simulink model "downsample_demo_tests"  (R2019b)
settings: Solver=FixedStepDiscrete  StartTime=0  StopTime=100  RelTol=1e-3
libraries: dspsigops x6
settings Model: Creator=cyarp  LastModifiedBy=cyarp

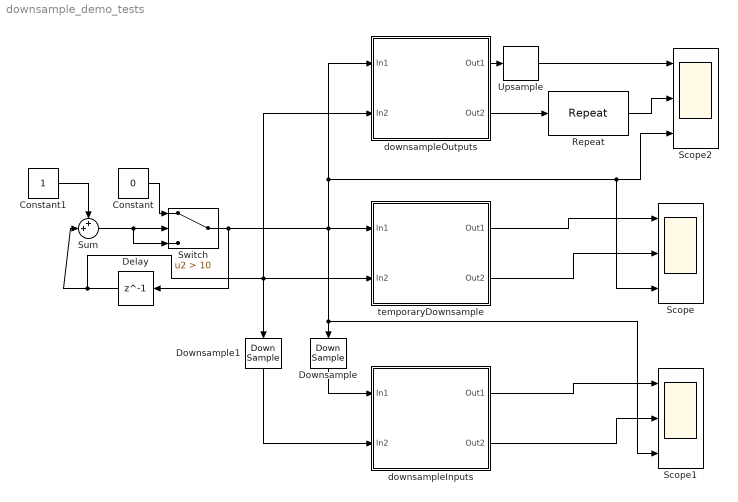
== system downsample_demo_tests ==
  Constant : Constant  Value=0  OutDataTypeStr=single
  Constant1 : Constant  OutDataTypeStr=single
  Delay : Delay  DelayLength=1  SampleTime=4
  Downsample : DownSample  N=4  RateOptions=Allow multirate processing
  Downsample1 : DownSample  N=4  RateOptions=Allow multirate processing
  Repeat : dspsigops/Repeat  N=4  InputProcessing=Columns as channels (frame based)  RateOptions=Allow multirate processing  ic=0  mode=Unused parameter value
      settings: SourceProductName=DSP System Toolbox
  Scope : Scope  NumInputPorts=3
  Scope1 : Scope  NumInputPorts=3
  Scope2 : Scope  NumInputPorts=3
  Sum : Sum  Inputs=++|
  Switch : Switch  Criteria=u2 > Threshold  Threshold=10
  Upsample : dspsigops/Upsample  N=4  phase=0  RateOptions=Allow multirate processing  ic=0  mode=Unused parameter value
  downsampleInputs : Subsystem
  downsampleOutputs : Subsystem
  temporaryDownsample : Subsystem
  wires:
  Delay/1 -> downsampleOutputs/2(In2), Downsample1/1, temporaryDownsample/2(In2), Sum/2
  Switch/1 -> Delay/1, temporaryDownsample/1(In1), downsampleOutputs/1(In1), Scope2/3, Scope/3, Scope1/3, Downsample/1
  Sum/1 -> Switch/2, Switch/3
  Constant/1 -> Switch/1
  Constant1/1 -> Sum/1
  temporaryDownsample/1(Out1) -> Scope/1
  temporaryDownsample/2(Out2) -> Scope/2
  downsampleInputs/1(Out1) -> Scope1/1
  downsampleInputs/2(Out2) -> Scope1/2
  Downsample1/1 -> downsampleInputs/2(In2)
  Downsample/1 -> downsampleInputs/1(In1)
  downsampleOutputs/1(Out1) -> Upsample/1
  downsampleOutputs/2(Out2) -> Repeat/1
  Upsample/1 -> Scope2/1
  Repeat/1 -> Scope2/2

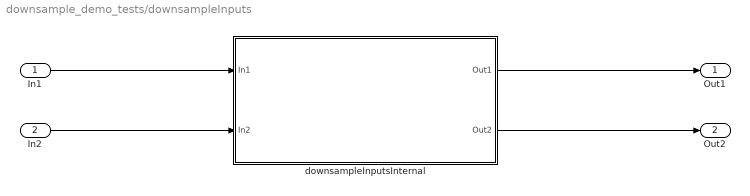
== system downsample_demo_tests/downsampleInputs ==
  In1 : Inport
  In2 : Inport  Port=2
  downsampleInputsInternal : Subsystem
  Out1 : Outport
  Out2 : Outport  Port=2
  wires:
  In1/1 -> downsampleInputsInternal/1(In1)
  In2/1 -> downsampleInputsInternal/2(In2)
  downsampleInputsInternal/1(Out1) -> Out1/1
  downsampleInputsInternal/2(Out2) -> Out2/1

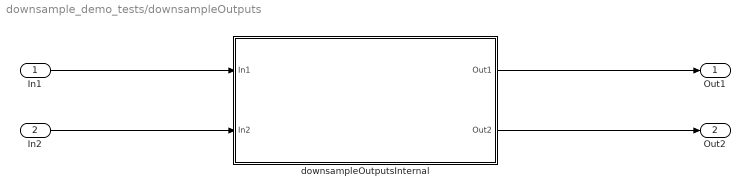
== system downsample_demo_tests/downsampleOutputs ==
  In1 : Inport
  In2 : Inport  Port=2
  downsampleOutputsInternal : Subsystem
  Out1 : Outport
  Out2 : Outport  Port=2
  wires:
  In1/1 -> downsampleOutputsInternal/1(In1)
  In2/1 -> downsampleOutputsInternal/2(In2)
  downsampleOutputsInternal/1(Out1) -> Out1/1
  downsampleOutputsInternal/2(Out2) -> Out2/1

== system downsample_demo_tests/temporaryDownsample ==
  In1 : Inport
  In2 : Inport  Port=2
  temporaryDownsampleInternal : Subsystem
  Out1 : Outport
  Out2 : Outport  Port=2
  wires:
  In1/1 -> temporaryDownsampleInternal/1(In1)
  In2/1 -> temporaryDownsampleInternal/2(In2)
  temporaryDownsampleInternal/1(Out1) -> Out1/1
  temporaryDownsampleInternal/2(Out2) -> Out2/1

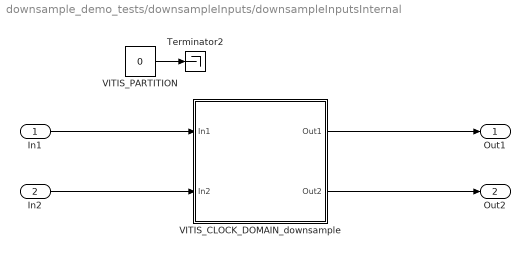
== system downsample_demo_tests/downsampleInputs/downsampleInputsInternal ==
  In1 : Inport
  In2 : Inport  Port=2
  Terminator2 : Terminator
  VITIS_CLOCK_DOMAIN_downsample : Subsystem
  VITIS_PARTITION : Constant  Value=0
  Out1 : Outport
  Out2 : Outport  Port=2
  wires:
  In1/1 -> VITIS_CLOCK_DOMAIN_downsample/1(In1)
  VITIS_CLOCK_DOMAIN_downsample/2(Out2) -> Out2/1
  In2/1 -> VITIS_CLOCK_DOMAIN_downsample/2(In2)
  VITIS_CLOCK_DOMAIN_downsample/1(Out1) -> Out1/1
  VITIS_PARTITION/1 -> Terminator2/1

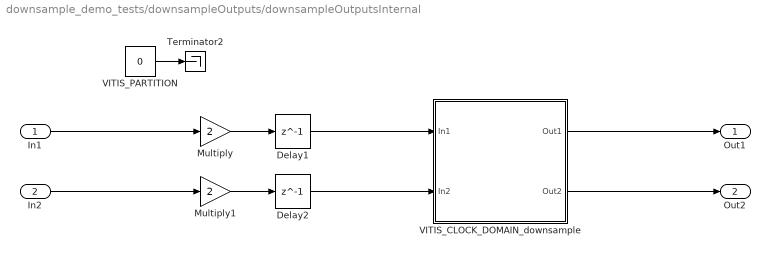
== system downsample_demo_tests/downsampleOutputs/downsampleOutputsInternal ==
  In1 : Inport
  In2 : Inport  Port=2
  Delay1 : Delay  DelayLength=1
  Delay2 : Delay  DelayLength=1
  Multiply : Gain  Gain=2
  Multiply1 : Gain  Gain=2
  Terminator2 : Terminator
  VITIS_CLOCK_DOMAIN_downsample : Subsystem
  VITIS_PARTITION : Constant  Value=0
  Out1 : Outport
  Out2 : Outport  Port=2
  wires:
  In1/1 -> Multiply/1
  In2/1 -> Multiply1/1
  Multiply1/1 -> Delay2/1
  Delay1/1 -> VITIS_CLOCK_DOMAIN_downsample/1(In1)
  VITIS_CLOCK_DOMAIN_downsample/2(Out2) -> Out2/1
  Multiply/1 -> Delay1/1
  Delay2/1 -> VITIS_CLOCK_DOMAIN_downsample/2(In2)
  VITIS_CLOCK_DOMAIN_downsample/1(Out1) -> Out1/1
  VITIS_PARTITION/1 -> Terminator2/1

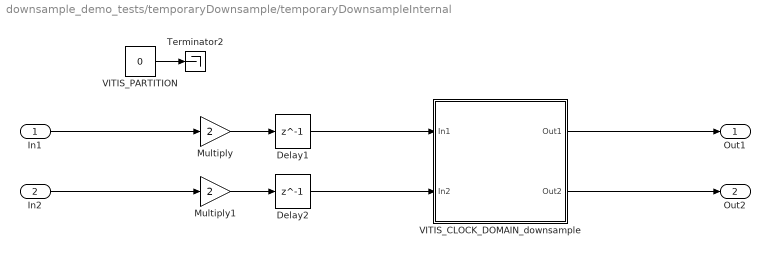
== system downsample_demo_tests/temporaryDownsample/temporaryDownsampleInternal ==
  In1 : Inport
  In2 : Inport  Port=2
  Delay1 : Delay  DelayLength=1
  Delay2 : Delay  DelayLength=1
  Multiply : Gain  Gain=2
  Multiply1 : Gain  Gain=2
  Terminator2 : Terminator
  VITIS_CLOCK_DOMAIN_downsample : Subsystem
  VITIS_PARTITION : Constant  Value=0
  Out1 : Outport
  Out2 : Outport  Port=2
  wires:
  In1/1 -> Multiply/1
  In2/1 -> Multiply1/1
  Multiply1/1 -> Delay2/1
  Delay1/1 -> VITIS_CLOCK_DOMAIN_downsample/1(In1)
  VITIS_CLOCK_DOMAIN_downsample/2(Out2) -> Out2/1
  Multiply/1 -> Delay1/1
  Delay2/1 -> VITIS_CLOCK_DOMAIN_downsample/2(In2)
  VITIS_CLOCK_DOMAIN_downsample/1(Out1) -> Out1/1
  VITIS_PARTITION/1 -> Terminator2/1

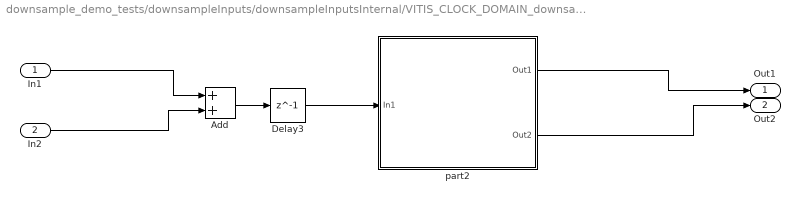
== system downsample_demo_tests/downsampleInputs/downsampleInputsInternal/VITIS_CLOCK_DOMAIN_downsample ==
  In1 : Inport
  In2 : Inport  Port=2
  Add : Sum
  Delay3 : Delay  DelayLength=1
  part2 : Subsystem
  Out1 : Outport
  Out2 : Outport  Port=2
  wires:
  Add/1 -> Delay3/1
  In2/1 -> Add/2
  In1/1 -> Add/1
  Delay3/1 -> part2/1(In1)
  part2/1(Out1) -> Out1/1
  part2/2(Out2) -> Out2/1

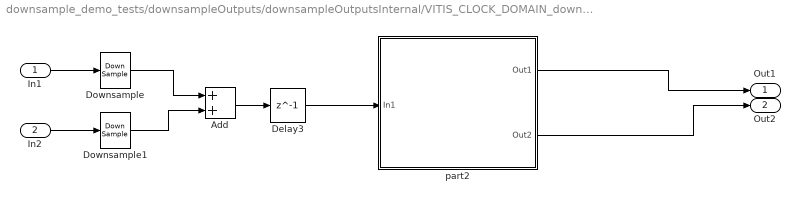
== system downsample_demo_tests/downsampleOutputs/downsampleOutputsInternal/VITIS_CLOCK_DOMAIN_downsample ==
  In1 : Inport
  In2 : Inport  Port=2
  Add : Sum
  Delay3 : Delay  DelayLength=1
  Downsample : DownSample  N=4  RateOptions=Allow multirate processing
  Downsample1 : DownSample  N=4  RateOptions=Allow multirate processing
  part2 : Subsystem
  Out1 : Outport
  Out2 : Outport  Port=2
  wires:
  Add/1 -> Delay3/1
  In2/1 -> Downsample1/1
  Downsample1/1 -> Add/2
  In1/1 -> Downsample/1
  Downsample/1 -> Add/1
  Delay3/1 -> part2/1(In1)
  part2/1(Out1) -> Out1/1
  part2/2(Out2) -> Out2/1

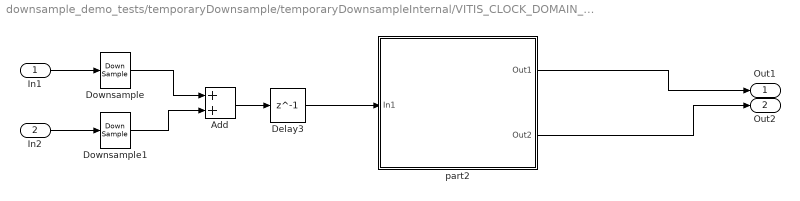
== system downsample_demo_tests/temporaryDownsample/temporaryDownsampleInternal/VITIS_CLOCK_DOMAIN_downsample ==
  In1 : Inport
  In2 : Inport  Port=2
  Add : Sum
  Delay3 : Delay  DelayLength=1
  Downsample : DownSample  N=4  RateOptions=Allow multirate processing
  Downsample1 : DownSample  N=4  RateOptions=Allow multirate processing
  part2 : Subsystem
  Out1 : Outport
  Out2 : Outport  Port=2
  wires:
  Add/1 -> Delay3/1
  In2/1 -> Downsample1/1
  Downsample1/1 -> Add/2
  In1/1 -> Downsample/1
  Downsample/1 -> Add/1
  Delay3/1 -> part2/1(In1)
  part2/1(Out1) -> Out1/1
  part2/2(Out2) -> Out2/1

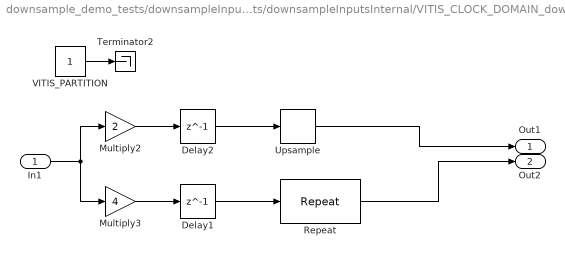
== system downsample_demo_tests/downsampleInputs/downsampleInputsInternal/VITIS_CLOCK_DOMAIN_downsample/part2 ==
  In1 : Inport
  Delay1 : Delay  DelayLength=1
  Delay2 : Delay  DelayLength=1
  Multiply2 : Gain  Gain=2
  Multiply3 : Gain  Gain=4
  Repeat : dspsigops/Repeat  N=4  InputProcessing=Columns as channels (frame based)  RateOptions=Allow multirate processing  ic=0  mode=Unused parameter value
      settings: SourceProductName=DSP System Toolbox
  Terminator2 : Terminator
  Upsample : dspsigops/Upsample  N=4  phase=0  RateOptions=Allow multirate processing  ic=0  mode=Unused parameter value
  VITIS_PARTITION : Constant
  Out1 : Outport
  Out2 : Outport  Port=2
  wires:
  Multiply2/1 -> Delay2/1
  Multiply3/1 -> Delay1/1
  Upsample/1 -> Out1/1
  Delay1/1 -> Repeat/1
  Delay2/1 -> Upsample/1
  Repeat/1 -> Out2/1
  In1/1 -> Multiply3/1, Multiply2/1
  VITIS_PARTITION/1 -> Terminator2/1

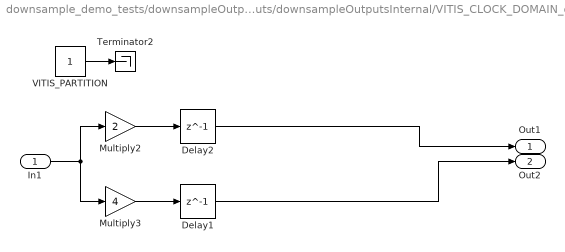
== system downsample_demo_tests/downsampleOutputs/downsampleOutputsInternal/VITIS_CLOCK_DOMAIN_downsample/part2 ==
  In1 : Inport
  Delay1 : Delay  DelayLength=1
  Delay2 : Delay  DelayLength=1
  Multiply2 : Gain  Gain=2
  Multiply3 : Gain  Gain=4
  Terminator2 : Terminator
  VITIS_PARTITION : Constant
  Out1 : Outport
  Out2 : Outport  Port=2
  wires:
  Multiply2/1 -> Delay2/1
  Multiply3/1 -> Delay1/1
  Delay2/1 -> Out1/1
  Delay1/1 -> Out2/1
  In1/1 -> Multiply3/1, Multiply2/1
  VITIS_PARTITION/1 -> Terminator2/1

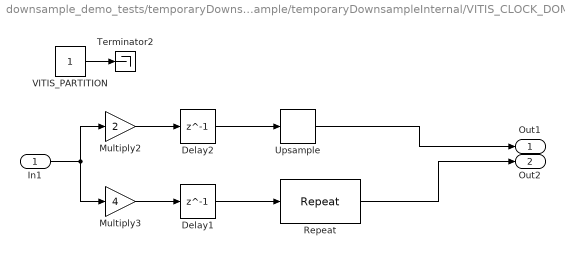
== system downsample_demo_tests/temporaryDownsample/temporaryDownsampleInternal/VITIS_CLOCK_DOMAIN_downsample/part2 ==
  In1 : Inport
  Delay1 : Delay  DelayLength=1
  Delay2 : Delay  DelayLength=1
  Multiply2 : Gain  Gain=2
  Multiply3 : Gain  Gain=4
  Repeat : dspsigops/Repeat  N=4  InputProcessing=Columns as channels (frame based)  RateOptions=Allow multirate processing  ic=0  mode=Unused parameter value
      settings: SourceProductName=DSP System Toolbox
  Terminator2 : Terminator
  Upsample : dspsigops/Upsample  N=4  phase=0  RateOptions=Allow multirate processing  ic=0  mode=Unused parameter value
  VITIS_PARTITION : Constant
  Out1 : Outport
  Out2 : Outport  Port=2
  wires:
  Multiply2/1 -> Delay2/1
  Multiply3/1 -> Delay1/1
  Upsample/1 -> Out1/1
  Delay1/1 -> Repeat/1
  Delay2/1 -> Upsample/1
  Repeat/1 -> Out2/1
  In1/1 -> Multiply3/1, Multiply2/1
  VITIS_PARTITION/1 -> Terminator2/1
